simulink model "testing3"  (R2021a)
settings: Solver=FixedStepDiscrete  StartTime=0.0  StopTime=50  FixedStep=1  RelTol=1e-3
libraries: simulink x3
settings Model: Creator=Rahul  LastModifiedBy=Rahul

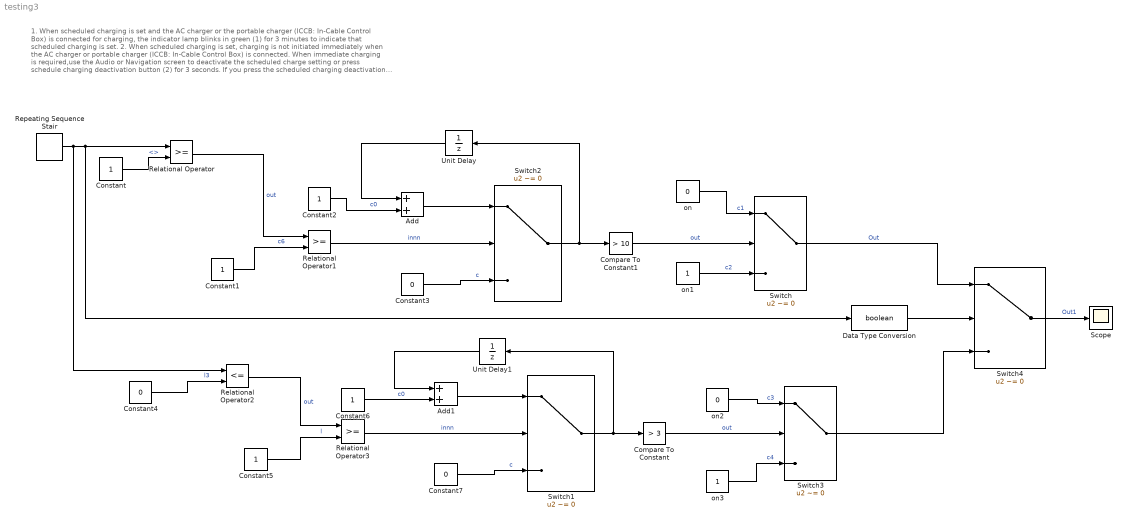
== system testing3 ==
  note: 1. When scheduled charging is set and the AC charger or the portable charger (ICCB: In-Cable Control Box) is connected for charging, the indicator lamp blinks in green (1) for 3 minutes to indicate that scheduled charging is set.
      | 2. When scheduled charging is set, charging is not initiated immediately when the AC charger or portable charger (ICCB: In-Cable Control Box) is connected. When immediate charging is required,use the Audio or Navigation screen to deactivate the scheduled charge setting
      | or press schedule charging deactivation button (2) for 3 seconds.
      | If you press the scheduled charging deactivation button (2) to immediately charge the battery,
      | charging must be initiated 3 minutes after the charging cable has been connected. When you press the scheduled charging deactivation button (2) for immediate charging, the scheduled charge setting
  Add : Sum
  Add1 : Sum
  Compare To Constant : simulink/Logic and Bit Operations/Compare To Constant  relop=>  const=3  OutDataTypeStr=boolean
  Compare To Constant1 : simulink/Logic and Bit Operations/Compare To Constant  relop=>  const=10  OutDataTypeStr=boolean
  Constant{,1..2,5..6} (5 alike) : Constant
  Constant3 : Constant  Value=0
  Constant4 : Constant  Value=0
  Constant7 : Constant  Value=0
  Data Type Conversion : DataTypeConversion  OutDataTypeStr=boolean
  Relational Operator : RelationalOperator  OutDataTypeStr=boolean  RndMeth=Simplest
  Relational Operator1 : RelationalOperator  OutDataTypeStr=boolean  RndMeth=Simplest
  Relational Operator2 : RelationalOperator  Operator=<=  OutDataTypeStr=boolean  RndMeth=Simplest
  Relational Operator3 : RelationalOperator  OutDataTypeStr=boolean  RndMeth=Simplest
  Repeating Sequence Stair : simulink/Sources/Repeating Sequence Stair  OutValues=[1 1 1 1 1 1 1 1 1 1 1 0 0 0 0 0]  tsamp=-1  OutMin=[]  OutMax=[]  OutDataTypeStr=double  OutputDataTypeScalingMode=double  OutDataType=fixdt(0,8)  ConRadixGroup=Best Precision: Vector-wise  OutScaling=2^-12
  Scope : Scope
  Switch : Switch  Criteria=u2 ~= 0  OutDataTypeStr=boolean
  Switch1 : Switch  Criteria=u2 ~= 0
  Switch2 : Switch  Criteria=u2 ~= 0
  Switch3 : Switch  Criteria=u2 ~= 0
  Switch4 : Switch  Criteria=u2 ~= 0  OutDataTypeStr=boolean
  Unit Delay : UnitDelay  SampleTime=-1  HasFrameUpgradeWarning=on
  Unit Delay1 : UnitDelay  SampleTime=-1  HasFrameUpgradeWarning=on
  on : Constant  Value=0  OutDataTypeStr=boolean
  on1 : Constant
  on2 : Constant  Value=0  OutDataTypeStr=boolean
  on3 : Constant
  wires:
  Relational Operator/1 -> Relational Operator1/1  "out"
  Constant/1 -> Relational Operator/2  "<>"
  Constant1/1 -> Relational Operator1/2  "c6"
  Switch2/1 -> Unit Delay/1, Compare To Constant1/1
  Relational Operator1/1 -> Switch2/2  "innn"
  Add/1 -> Switch2/1
  Constant3/1 -> Switch2/3  "c"
  Compare To Constant1/1 -> Switch/2  "out"
  Constant2/1 -> Add/2  "c0"
  Unit Delay/1 -> Add/1
  on/1 -> Switch/1  "c1"
  Switch/1 -> Switch4/1  "Out"
  on1/1 -> Switch/3  "c2"
  Relational Operator2/1 -> Relational Operator3/1  "out"
  Constant4/1 -> Relational Operator2/2  "l3"
  Constant5/1 -> Relational Operator3/2  "l"
  Constant6/1 -> Add1/2  "c0"
  Constant7/1 -> Switch1/3  "c"
  Add1/1 -> Switch1/1
  Unit Delay1/1 -> Add1/1
  Switch1/1 -> Unit Delay1/1, Compare To Constant/1
  Relational Operator3/1 -> Switch1/2  "innn"
  Compare To Constant/1 -> Switch3/2  "out"
  on2/1 -> Switch3/1  "c3"
  on3/1 -> Switch3/3  "c4"
  Switch3/1 -> Switch4/3
  Switch4/1 -> Scope/1  "Out1"
  Repeating Sequence Stair/1 -> Relational Operator2/1, Data Type Conversion/1, Relational Operator/1
  Data Type Conversion/1 -> Switch4/2
